simulink model "model06c"  (R2018b)
settings: Solver=ode4  StartTime=0.0  StopTime=10  FixedStep=0.01  RelTol=1e-3
values from neighbouring files (symbols this model uses):
  A_sys = [  0   1 ... (first row only)    [main.m]
  b = 1    [data.m]
  B_sys = [B1_sys B2_sys]    [main.m]
  C_sys = [1 0]    [main.m]
  D = m_br*a_br*h_br    (= 44.002512)    [data.m]
  D_sys = [0 a5]    [main.m]
  g = 9.81    [data.m]
  h_br = 1.028    [data.m]
  h_r = (h_br*m_br - m_b*h_b)/m_r    (= 1.09984)    [data.m]
  J_br = m_br * h_br^2    (= 91.940208)    [data.m]
  J_r = m_r * h_r^2    (= 90.72360192)    [data.m]
  k1 = b^2/((V^2*sin(lambda)-b*g*cos(lambda))*m_br*a_br*c*sin(lambda))    [main.m]
  k2 = b*g/(V^2*sin(lambda)-b*g*cos(lambda))    [main.m]
  m_br = m_b + m_r    (= 87)    [data.m]
  m_r = 75    [data.m]
  V = 4    [data.m]
  x_init = T^-1*init_conds(2, :)'    [main.m]
undefined symbols (not defined in the file or in its folder): K
settings Model: Creator=franc  LastModifiedBy=franc

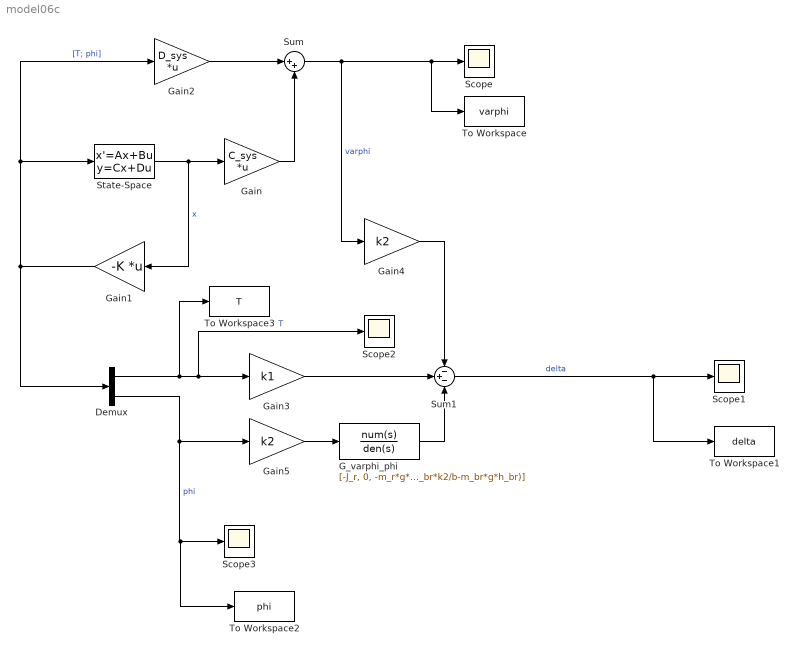
== system model06c ==
  Demux : Demux  Outputs=2
  G_varphi_phi : TransferFcn  Numerator=[-J_r, 0, -m_r*g*h_r]  Denominator=[J_br, D*V*k2/b, (m_br*V^2*h_br*k2/b-m_br*g*h_br)]
  Gain : Gain  Gain=C_sys  Multiplication=Matrix(K*u)
  Gain1 : Gain  Gain=-K  Multiplication=Matrix(K*u)
  Gain2 : Gain  Gain=D_sys  Multiplication=Matrix(K*u)
  Gain3 : Gain  Gain=k1
  Gain4 : Gain  Gain=k2
  Gain5 : Gain  Gain=k2
  Scope{,1..3} (4 alike) : Scope
  State-Space : StateSpace  A=A_sys  B=B_sys  C=eye(2)  D=zeros(2, 2)  InitialCondition=x_init
  Sum : Sum  Inputs=|++
  Sum1 : Sum  Inputs=-+-
  To Workspace : ToWorkspace  VariableName=varphi  SaveFormat=Timeseries  SampleTime=-1
  To Workspace1 : ToWorkspace  VariableName=delta  SaveFormat=Timeseries  SampleTime=-1
  To Workspace2 : ToWorkspace  VariableName=phi  SaveFormat=Timeseries  SampleTime=-1
  To Workspace3 : ToWorkspace  VariableName=T  SaveFormat=Timeseries  SampleTime=-1
  wires:
  State-Space/1 -> Gain1/1, Gain/1  "x"
  Gain1/1 -> Demux/1, State-Space/1, Gain2/1  "[T; phi]"
  Gain/1 -> Sum/2
  Gain2/1 -> Sum/1
  Sum/1 -> To Workspace/1, Scope/1, Gain4/1  "varphi"
  Demux/1 -> To Workspace3/1, Scope2/1, Gain3/1  "T"
  Gain3/1 -> Sum1/2
  Gain4/1 -> Sum1/1
  Sum1/1 -> To Workspace1/1, Scope1/1  "delta"
  Demux/2 -> To Workspace2/1, Scope3/1, Gain5/1  "phi"
  Gain5/1 -> G_varphi_phi/1
  G_varphi_phi/1 -> Sum1/3
